simulink model "sampleModel308"  (R2021b)
settings: Solver=VariableStepAuto  StartTime=0.0  StopTime=10.0  RelTol=1e-3
libraries: simulink x1
settings Model: Creator=user  LastModifiedBy=user

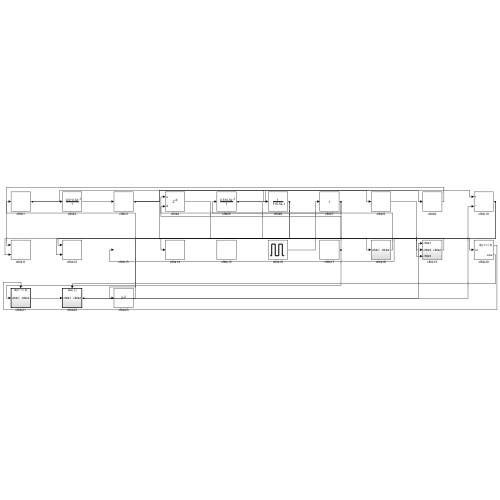
[thumbnail: Simulink's stored preview of the top-level diagram]
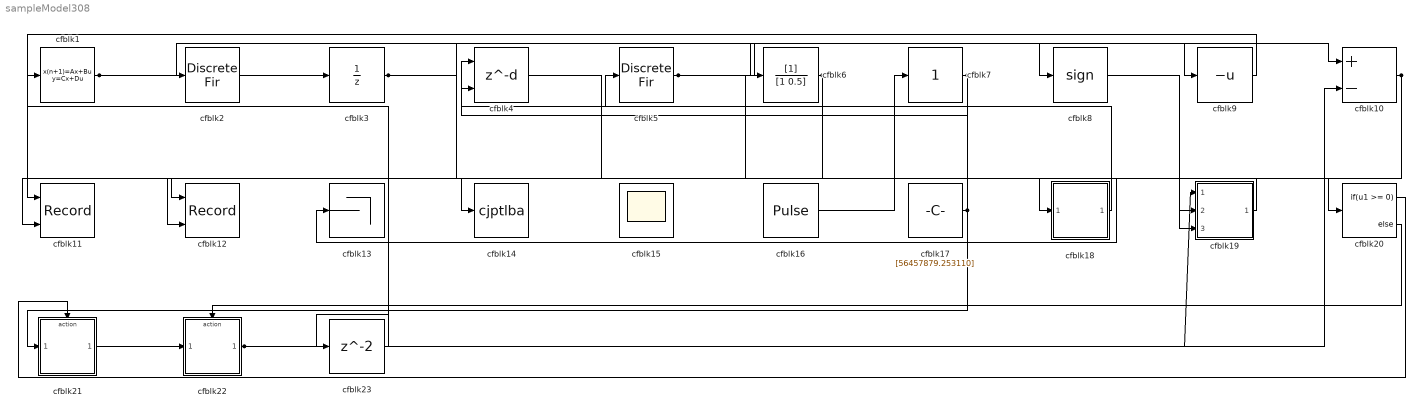
== system sampleModel308 ==
  cfblk1 : DiscreteStateSpace
  cfblk10 : Sum  Inputs=+-
  cfblk11 : Record  FileSettingsInternal="{\"entries\":[{\"content\":{\"excelSettings\":{\"content\":{},\"type\":\"Streamout.ExcelSettings\"}},\"type\":\"Streamout.FileSettingStorage\",\"uuid\":\"453004bc-ad0f-4aa7-8e95-8703dcf3554b\"}],\"packageUris\":[\"http://schema.mathworks.com/mf0/streamout_blocks/R2020a\"],\"version\":\"1.0\"}"  Layout=[1 1]  SignalsInternal="{\"entries\":[{\"content\":{\"signals\":[{\"content\":{\"blockPath\":[\"sampleModel308/cfblk11\"],\"channel\":[],\"dimensions\":[1],\"domain\":\"sampleModel308/cfblk11\",\"lineColor\":\"#a2142f\",\"plots\":[1],\"port\":1,\"sid\":[\"\"],\"signalID\":13072,\"signalName\":\"cfblk9\"},\"type\":\"RecordBlkView.Signal\",\"uuid\":\"db24b52a-3bb6-44ec-8338-eb2f70d47c8d\"},{\"content\":{\"blockPath\":[\"sampleModel308/cfblk11\"],\"channel\":[],\"dimensions\":[1],\"domain\":\"sampleModel308/cfblk11\",\"lineColor\":\"#139fff\",\"plots\":[1],\"port\":2,\"sid\":[\"\"],\"signalID\":13076,\"signalName\":\"cfblk7\"},\"type\":\"RecordBlkView.Signal\",\"uuid\":\"4eaa3d7c-6306-46cf-8424-7c8e57f0c991\"}]},\"type\":\"RecordBlkView.InputSignals\",\"uuid\":\"8a6803a5-0933-459b-a850-a5a5caa3608e\"}],\"packageUris\":[\"http://schema.mathworks.com/mf0/streamout_blocks/R2020a\"],\"version\":\"1.0\"}"  VisualizationBindings="{\"xyplotplugin\":{\"info\":[{\"series\":[{\"bindingParametersList\":[{\"parameter\":\"X-Axis\",\"signalID\":13072,\"signalName\":\"cfblk9\"},{\"parameter\":\"Y-Axis\",\"signalID\":13076,\"signalName\":\"cfblk7\"}],\"seriesID\":30220}],\"subplotID\":1}]}}"  CompatibilityTag=XY
  cfblk12 : Record  FileSettingsInternal="{\"entries\":[{\"content\":{\"excelSettings\":{\"content\":{},\"type\":\"Streamout.ExcelSettings\"}},\"type\":\"Streamout.FileSettingStorage\",\"uuid\":\"d919508d-cbf9-41ae-87c2-c061d7f31b3e\"}],\"packageUris\":[\"http://schema.mathworks.com/mf0/streamout_blocks/R2020a\"],\"version\":\"1.0\"}"  Layout=[1 1]  SignalsInternal="{\"entries\":[{\"content\":{\"signals\":[{\"content\":{\"blockPath\":[\"sampleModel308/cfblk12\"],\"channel\":[],\"dimensions\":[1],\"domain\":\"sampleModel308/cfblk12\",\"lineColor\":\"#a2142f\",\"plots\":[1],\"port\":1,\"sid\":[\"\"],\"signalID\":13080,\"signalName\":\"cfblk10\"},\"type\":\"RecordBlkView.Signal\",\"uuid\":\"1ab5bd5c-1e83-451e-8082-1dc5e620c8aa\"},{\"content\":{\"blockPath\":[\"sampleModel308/cfblk12\"],\"channel\":[],\"dimensions\":[1],\"domain\":\"sampleModel308/cfblk12\",\"lineColor\":\"#139fff\",\"plots\":[1],\"port\":2,\"sid\":[\"\"],\"signalID\":13084,\"signalName\":\"cfblk6\"},\"type\":\"RecordBlkView.Signal\",\"uuid\":\"ae4597d2-a46a-407c-8dd9-f901ddb3e1bd\"}]},\"type\":\"RecordBlkView.InputSignals\",\"uuid\":\"c57f3ff0-5206-4594-a678-462aff14e986\"}],\"packageUris\":[\"http://schema.mathworks.com/mf0/streamout_blocks/R2020a\"],\"version\":\"1.0\"}"  VisualizationBindings="{\"xyplotplugin\":{\"info\":[{\"series\":[{\"bindingParametersList\":[{\"parameter\":\"X-Axis\",\"signalID\":13080,\"signalName\":\"cfblk10\"},{\"parameter\":\"Y-Axis\",\"signalID\":13084,\"signalName\":\"cfblk6\"}],\"seriesID\":34583}],\"subplotID\":1}]}}"  CompatibilityTag=XY
  cfblk13 : Terminator
  cfblk14 : ToWorkspace  VariableName=cjptlba  SaveFormat=Timeseries  SampleTime=-1
  cfblk15 : Scope
      settings: Floating=on
  cfblk16 : DiscretePulseGenerator  PulseType=Time based  Amplitude=[-535886736.499142]  Period=[98663836.221798]  PulseWidth=5  PhaseDelay=[4.000000]
  cfblk17 : Constant  Value=[56457879.253110]  SampleTime=1
  cfblk18 : Subsystem
  cfblk19 : Subsystem
  cfblk2 : DiscreteFir  SampleTime=1
  cfblk20 : If  IfExpression=u1 >= 0  SampleTime=1
  cfblk21 : Subsystem  TreatAsAtomicUnit=on
  cfblk22 : Subsystem  TreatAsAtomicUnit=on
  cfblk23 : Delay  SampleTime=1
  cfblk3 : UnitDelay  HasFrameUpgradeWarning=on
  cfblk4 : Delay  DelayLengthSource=Input port  SampleTime=1
      settings: InputPortMap=u0,p1
  cfblk5 : DiscreteFir  SampleTime=1
  cfblk6 : DiscreteFilter  SampleTime=1
  cfblk7 : simulink/Math Operations/Slider Gain  gain=1  low=0  high=2
  cfblk8 : Signum
  cfblk9 : UnaryMinus
  wires:
  cfblk18/1(cfblk2) -> cfblk5/1
  cfblk1/1 -> cfblk9/1, cfblk2/1
  cfblk17/1 -> cfblk4/1, cfblk21/1(cfblk1)
  cfblk21/1(cfblk2) -> cfblk22/1(cfblk1)
  cfblk7/1 -> cfblk4/2, cfblk11/2
  cfblk10/1 -> cfblk13/1, cfblk12/1
  cfblk2/1 -> cfblk3/1
  cfblk16/1 -> cfblk7/1
  cfblk19/1(cfblk2) -> cfblk14/1
  cfblk4/1 -> cfblk18/1(cfblk1)
  cfblk22/1(cfblk2) -> cfblk19/1(cfblk1), cfblk10/2
  cfblk8/1 -> cfblk19/2(cfblk4)
  cfblk9/1 -> cfblk11/1
  cfblk5/1 -> cfblk8/1, cfblk20/1
  cfblk3/1 -> cfblk19/3(cfblk5), cfblk6/1, cfblk10/1
  cfblk6/1 -> cfblk12/2, cfblk23/1
  cfblk20/1 -> cfblk21/Action
  cfblk20/2 -> cfblk22/Action
  cfblk23/1 -> cfblk1/1

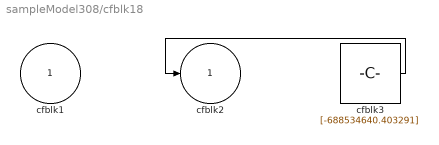
== system sampleModel308/cfblk18 ==
  cfblk1 : Inport
  cfblk3 : Constant  Value=[-688534640.403291]  SampleTime=1
  cfblk2 : Outport
  wires:
  cfblk3/1 -> cfblk2/1

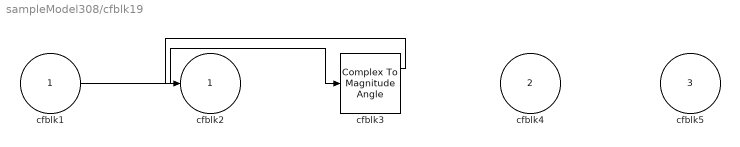
== system sampleModel308/cfblk19 ==
  cfblk1 : Inport
  cfblk4 : Inport  Port=2
  cfblk5 : Inport  Port=3
  cfblk3 : ComplexToMagnitudeAngle
  cfblk2 : Outport
  wires:
  cfblk1/1 -> cfblk3/1
  cfblk3/1 -> cfblk2/1

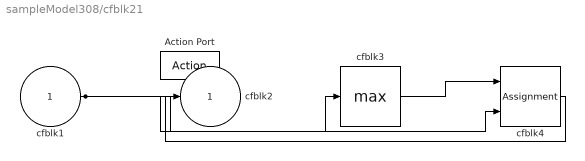
== system sampleModel308/cfblk21 ==
  cfblk1 : Inport
  Action Port : ActionPort  ActionPortLabel=if(u1 >= 0)
  cfblk3 : MinMax  Function=max
  cfblk4 : Assignment  DiagnosticForDimensions=Warning  IndexOptions=Index vector (dialog)  Indices=1  OutputSizes=1
  cfblk2 : Outport
  wires:
  cfblk1/1 -> cfblk3/1, cfblk4/2
  cfblk4/1 -> cfblk2/1
  cfblk3/1 -> cfblk4/1

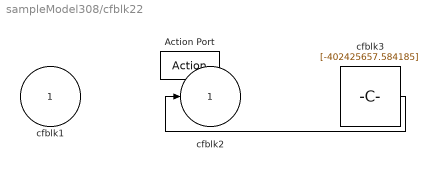
== system sampleModel308/cfblk22 ==
  cfblk1 : Inport
  Action Port : ActionPort  ActionPortLabel=else
  cfblk3 : Constant  Value=[-402425657.584185]  SampleTime=1
  cfblk2 : Outport
  wires:
  cfblk3/1 -> cfblk2/1
